simulink model "selft_of_q2x2sim"  (R2025b)
settings: Solver=ode45  StartTime=0.0  StopTime=15  MaxStep=.1  RelTol=1e-4
values from neighbouring files (symbols this model uses):
  A = zeros(sum(neqs), 4*NK)    [kernelsc.m]    (also in kernelscinv.m; kernelso.m; kernelsoinv.m; q2x2simu.m = zeros(2*xg))
  Ao = A - [P1; P2]*C    [q2x2simu.m]
  B = zeros(2*xg, 1)    [q2x2simu.m]
  Bo = [[P1; P2] + r*B, B]    [q2x2simu.m]
  C = B'    [q2x2simu.m]
  param = [a0, C1, Cth, Cp, Kq, M2, Cetm]    [bounds.m]
  qparam = [M, Omega, T, mu0, Delta]    [bounds.m]
  xg = 128    [bounds.m]    (also in q2x2simu.m)
  z0 = [p * v0_ic(x1); v0_ic(x0)]    [histogrametc.m]    (also in q2x2simu.m = [p*v0(x1), v0(x0)]')
  z0hat = 1.5 * z0    [histogrametc.m]    (also in q2x2simu.m = 1.5*z0)
undefined symbols (not defined in the file or in its folder): K1, K2
settings Model: Creator=humaloja  LastModifiedBy=koudohodeflorent

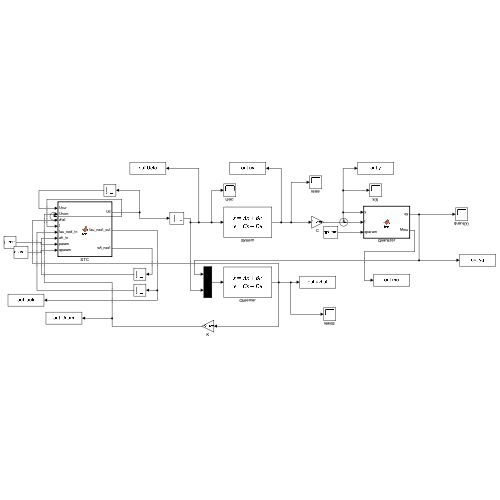
[thumbnail: Simulink's stored preview of the top-level diagram]
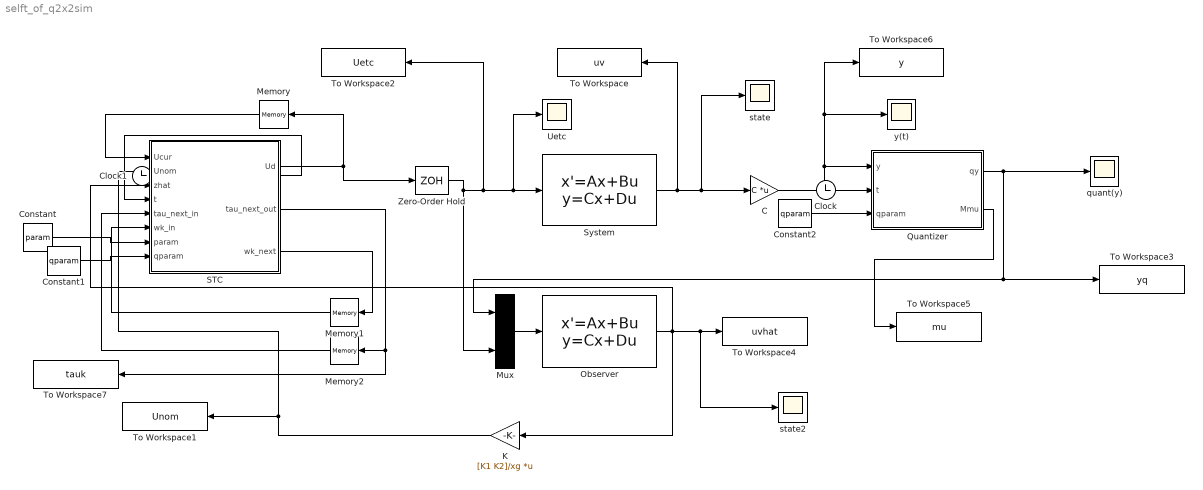
== system selft_of_q2x2sim ==
  C : Gain  Gain=C  Multiplication=Matrix(K*u) (u vector)
  Clock : Clock
  Clock1 : Clock
  Constant : Constant  Value=param  VectorParams1D=off
  Constant1 : Constant  Value=qparam  VectorParams1D=off
  Constant2 : Constant  Value=qparam  VectorParams1D=off
  K : Gain  Gain=[K1 K2]/xg  Multiplication=Matrix(K*u) (u vector)
  Memory : Memory
  Memory1 : Memory
  Memory2 : Memory
  Mux : Mux  Inputs=2
  Observer : StateSpace  A=Ao  B=Bo  C=eye(2*xg)  D=zeros(2*xg,2)  InitialCondition=z0hat
  Quantizer : MATLAB Function  TreatAsAtomicUnit=on
  STC : MATLAB Function  TreatAsAtomicUnit=on
  System : StateSpace  A=A  B=B  C=eye(2*xg)  D=zeros(2*xg,1)  InitialCondition=z0
  To Workspace : ToWorkspace  VariableName=uv  SaveFormat=Timeseries  SampleTime=-1
  To Workspace1 : ToWorkspace  VariableName=Unom  SaveFormat=Timeseries  SampleTime=-1
  To Workspace2 : ToWorkspace  VariableName=Uetc  SaveFormat=Timeseries  SampleTime=-1
  To Workspace3 : ToWorkspace  VariableName=yq  SaveFormat=Timeseries  SampleTime=-1
  To Workspace4 : ToWorkspace  VariableName=uvhat  SaveFormat=Timeseries  SampleTime=-1
  To Workspace5 : ToWorkspace  VariableName=mu  SaveFormat=Timeseries  SampleTime=-1
  To Workspace6 : ToWorkspace  VariableName=y  SaveFormat=Timeseries  SampleTime=-1
  To Workspace7 : ToWorkspace  VariableName=tauk  SaveFormat=Timeseries  SampleTime=-1
  Uetc : Scope
      settings: ActiveDisplayYMinimum=-18.44375  ActiveDisplayYMaximum=11.5145
  Zero-Order Hold : ZeroOrderHold  SampleTime=-1
  quant(y) : Scope
      settings: ActiveDisplayYMinimum=-10.5  ActiveDisplayYMaximum=4.5  DataLoggingVariableName=ScopeData2
  state : Scope
      settings: ActiveDisplayYMinimum=-5.0111601734068E+8  ActiveDisplayYMaximum=5.567956859341E+7  DataLoggingVariableName=ScopeData4
  state2 : Scope
      settings: ActiveDisplayYMinimum=-20.70698  ActiveDisplayYMaximum=18.96744
  y(t) : Scope
      settings: ActiveDisplayYMinimum=-1  ActiveDisplayYMaximum=1
  wires:
  Mux/1 -> Observer/1
  System/1 -> To Workspace/1, state/1, C/1
  Quantizer/1(qy) -> To Workspace3/1, Mux/1, quant(y)/1
  Clock/1 -> Quantizer/2(t)
  Observer/1 -> K/1, STC/3(zhat), state2/1, To Workspace4/1
  Zero-Order Hold/1 -> To Workspace2/1, Uetc/1, System/1, Mux/2
  C/1 -> To Workspace6/1, y(t)/1, Quantizer/1(y)
  Quantizer/2(Mmu) -> To Workspace5/1
  K/1 -> STC/2(Unom), To Workspace1/1
  Memory/1 -> STC/1(Ucur)
  Clock1/1 -> STC/4(t)
  STC/2(tau_next_out) -> To Workspace7/1, Memory2/1
  Memory2/1 -> STC/5(tau_next_in)
  STC/1(Ud) -> Memory/1, Zero-Order Hold/1
  STC/3(wk_next) -> Memory1/1
  Memory1/1 -> STC/6(wk_in)
  Constant1/1 -> STC/8(qparam)
  Constant/1 -> STC/7(param)
  Constant2/1 -> Quantizer/3(qparam)

== matlab function selft_of_q2x2sim/Quantizer ==
  data: y input; qy output; t input; Mmu output; qparam input
function [qy, Mmu] = fcn(y,t,qparam)
% parameters
M      = qparam(1);
Omega  = qparam(2);
T      = qparam(3);
mu0    = qparam(4);
Delta  = qparam(5);
% mu
mu = mu0*Omega^floor(t/T);
Mmu = M*mu;
% quantizer
if y/mu > M
  qy = M;
elseif y/mu < -M
  qy = -M;
else
  qy = Delta*floor(y/(mu*Delta) + 0.5);
end
% multiply output by mu
qy = mu*qy;

% FOR TESTING: disable quantization by just returning y
%qy = y;
end

== matlab function selft_of_q2x2sim/STC ==
  settings: updateMethod=DISCRETE
  data: Ucur input; Unom input; zhat input; Ud output; t input; tau_next_in input; tau_next_out output; wk_in input; wk_next output; param input; qparam input
function [Ud, tau_next_out, wk_next] = fcn(Ucur, Unom, zhat, t, tau_next_in, wk_in, param, qparam)
% STC  -  Self-Triggering Controller
% Constants from bounds.m  
a0   = param(1);    % double(abs(subs(Nb,z,1)*b(1)))
C1   = param(2);    % double(max([C2,C3]))
Cth  = param(3);    % Lyapunov gain 
Cp   = param(4);    % coupling constant
Kq   = param(5);  % P1/a(1) + (1+|p|)*(|r|+P2/b(1))
M2   = param(6);   % min([1/(1+Pbar), 1/(1+Lbar)])
Cetm = param(7);

% Design parameters  (must be identical to bounds.m)
M      = qparam(1);
Omega  = qparam(2);
T      = qparam(3);
mu0    = qparam(4);
delta  = -log(Omega)/T;   
Delta  = qparam(5);
xg = numel(zhat)/2;
% Self-triggering law
if t >= tau_next_in
    % ---- TRIGGER EVENT ----
    Ud = Unom;   % broadcast new control
    % A_k(w_k)
    Ak_val = Cth*C1*wk_in+ (Cp + Cth*C1)*(M2*M/(Omega*exp(delta*T)) + (1+Kq)*Delta)*mu0;
    % Next inter-event interval  (paper formula, corrected)
    dt = min(T,1/max(a0, C1*Cth) * log((1 + sqrt(1 + 4*a0*Cetm*wk_in/Ak_val))/2));
    tau_next_out = t + dt;
    wk_next = norm(zhat(1:xg),inf)+ norm(zhat(xg+1:2*xg), inf);
else
    % ---- HOLD ----
    Ud           = Ucur;
    tau_next_out = tau_next_in;
    wk_next = wk_in;
end
